simulink model "BackboneTracker"  (R2024b)
settings: Solver=ode4  StartTime=0.0  StopTime=inf  FixedStep=settings.samplingTime_s  MaxStep=1e-2  RelTol=1e-5
PostLoadFcn:
  | , if any(exist('dsrtsu_mdlpostloadfcn', 'file') ~= 0), dsrtsu_mdlpostloadfcn('Execute', bdroot); end,
  | , if any(exist('dsrtsu_mdlpostloadfcn', 'file') ~= 0), dsrtsu_mdlpostloadfcn('Execute', bdroot); end,
InitFcn:
  | , if any(exist('rtifpga_mdlclblib', 'file') ~= 0), rtifpga_mdlclblib('Init', bdroot); end,
values from neighbouring files (symbols this model uses):
  linearModalFrequency_Hz = linearPlantFrequency_Hz    [checkSettingsBackboneTracker.m]
  linearPhiEx = linearPlantPhiEx    [checkSettingsBackboneTracker.m]
undefined symbols (not defined in the file or in its folder): settings
libraries: simulink x8, dspswit3 x4, slpidlib x2, dspsigops x2
settings Model: Tag=RTI1202  DSRTSU_INTERNAL_RTIFPGA=200  DSRTSU_INTERNAL_RTI_TYPE=rti1202  DSRTSU_INTERNAL_RTI_VER=610  RTICANMMDATA=struct('GeneralSetupData',struct('modelroot','C:\UNI\Master\04_MA\05_Experiments','generalsettings',struct('filesettings',struct('destfolder',struct('Name','RTICANMM_FILES','Check',1),'buildfolder',struct('Name','.','Check',1),'AbsDestfolder',struct('Name','C:\UNI\Master\04_MA\05_Experiments\RTICANMM_FILES'),'AbsBuildfolder',struct('Name','C:\UNI\Master\04_MA\05_Experiments'))),'options',struct('addpaths',1,'rmpaths',1,'addtrcexclusion',true,'cannavigator',struct('checkmonitoring',0),'show_usrtrc',0,'use_usrtrc',0),'advanced',struct('options',ones(1,100)),'MPSetup',{{}},'RTI',struct('Type','RTI1202','Ver','7.13','Date','02-Nov-2019'),'modelname','PLL_autoStep_r2019b_rti','block','PLL_autoStep_r2019b_rti'))  DSRTSU_INTERNAL_RTISTBM_VER=22.2  Creator=patri  LastModifiedBy=phippold
settings SolverCC: AlgebraicLoopSolver=TrustRegion
settings DataIOCC: SaveOutput=off  SaveTime=off  ReturnWorkspaceOutputs=off
settings OptimizationCC: BlockReduction=off  OptimizeBlockIOStorage=off  BufferReuse=off  GlobalBufferReuse=off  ExpressionFolding=off  LocalBlockOutputs=off
settings DebuggingCC: UnconnectedInputMsg=warning  UnconnectedOutputMsg=warning  UnconnectedLineMsg=warning  ArithmeticOperatorsInVariantConditions=warning
settings HardwareCC: ProdBitPerPointer=32  ProdBitPerSizeT=32  ProdBitPerPtrDiffT=32  ProdLargestAtomicInteger=Integer  ProdEndianess=BigEndian  ProdWordSize=32  ProdHWDeviceType=Custom Processor->Custom  TargetIntDivRoundTo=Zero  TargetEndianess=BigEndian  TargetHWDeviceType=Custom Processor->Custom
settings ModelReferenceCC: EnableRefExpFcnMdlSchedulingChecks=on  ModelReferenceNumInstancesAllowed=Single  ModelReferenceMinAlgLoopOccurrences=on
settings SFSimCC: SimUseLocalCustomCode=off  MATLABDynamicMemAlloc=off  CustomCodeUndefinedFunction=UseInterfaceOnly
settings RTWCC: Description=dSPACE DS1202 Hardware Platform  SystemTargetFile=rti1202.tlc  MakeCommand=make_rti  TemplateMakefile=rti1202.tmf  RTWUseLocalCustomCode=off  GPUComputeCapability=3.5  DLArmComputeVersion=19.05
settings CodeAppCC: MaxIdLength=63  StateflowObjectComments=on
settings STFCustomTargetCC: ParMdlRefBuildCompliant=on  SystemTargetFile=rti1202.tlc
settings GRTTargetCC: TargetLangStandard=C89/C90 (ANSI)  CompOptLevelCompliant=off  ConcurrentExecutionCompliant=off  CombineOutputUpdateFcns=off  MatFileLogging=off  CPPClassGenCompliant=off  UseToolchainInfoCompliant=off
settings ConfigComp: CovMetricSettings=dswe
settings SimscapeCC: SimscapeNormalizeSystem=off

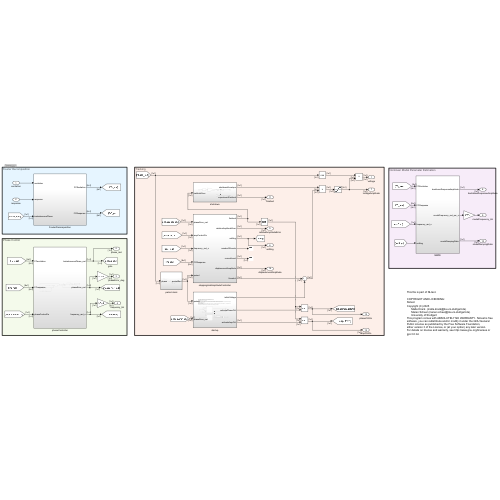
[thumbnail: Simulink's stored preview of the top-level diagram]
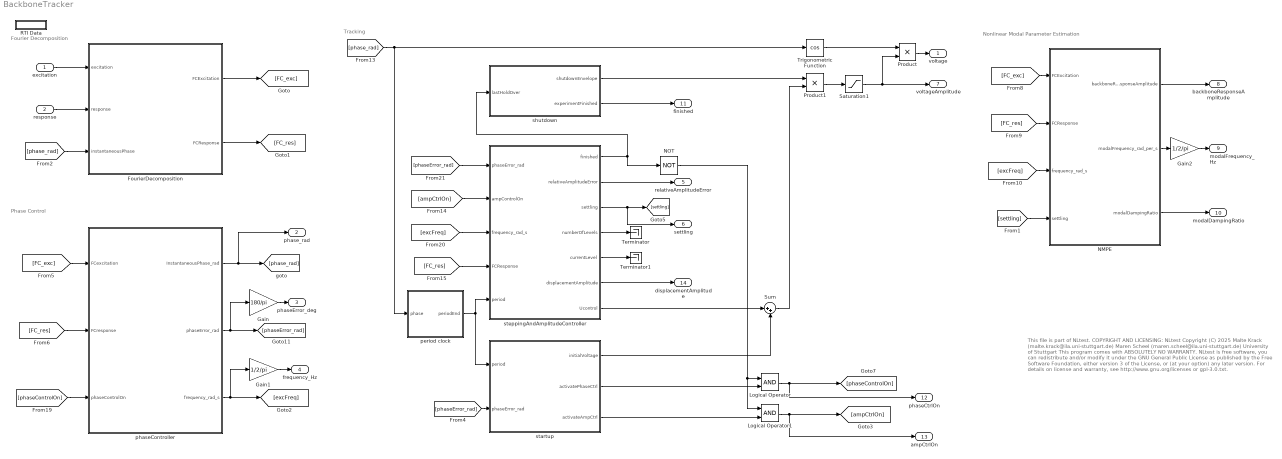
== system BackboneTracker ==
  note: Nonlinear Modal Parameter Estimation
  note: Phase Control
  note: Fourier Decomposition
  note: Tracking
  note: This file is part of NLtest.
      |
      | COPYRIGHT AND LICENSING:
      | NLtest
      | Copyright (C) 2025
      | Malte Krack (malte.krack@ila.uni-stuttgart.de)
      | Maren Scheel (maren.scheel@ila.uni-stuttgart.de)
      | University of Stuttgart
      | This program comes with ABSOLUTELY NO WARRANTY. NLtest is free software, you can redistribute and/or modify it under the GNU General Public License as published by the Free Software Foundation,
      | either version 3 of the License, or (at your option) any later version.
      | For details on license and warranty, see http://www.gnu.org/licenses or gpl-3.0.txt.
  excitation : Inport  OutDataTypeStr=double  PortDimensions=1
  response : Inport  Port=2  OutDataTypeStr=double  PortDimensions=1
  FourierDecomposition : Subsystem
  Gain : Gain  Gain=180/pi
  Gain1 : Gain  Gain=1/2/pi
  Gain2 : Gain  Gain=1/2/pi
  Logical Operator : Logic  AllPortsSameDT=off  OutDataTypeStr=boolean
  Logical Operator1 : Logic  AllPortsSameDT=off  OutDataTypeStr=boolean
  NMPE : Subsystem
  NOT : Logic  Operator=NOT  AllPortsSameDT=off  OutDataTypeStr=boolean
  Product : Product
  Product1 : Product
  RTI Data : Subsystem  Tag=struct('RTIDataServer',struct('RTIDataServerVs','2','RTIModelDescription','struct(''main'',''BackboneTracker_R2022a'',''sub'',''BackboneTracker_R2022a'',''isMp'',0)'))  LoadFcn="if exist('rtidc'), try,  rtidc('DataHostBlockClbLoad', gcbh); catch, disp(['Warning: ''LoadFcn'' for RTI Data block failed: ' lasterr]); end, end,"  mask(RTI_DATA_HOST){}
      mask help:
      | RTI Data Block.
      | This block is used by RTI to store internal model-dependent data.
      | Please keep this block on the root level of the model. Deleting this block will result in data loss.
      |
      | NEVER DELETE OR COPY THIS BLOCK!
      settings: CopyFcn="if exist('rtidc'), try,  rtidc('DataHostBlockClbCopy', gcbh); catch, disp(['Warning: ''CopyFcn'' for RTI Data block failed: ' lasterr]); end, end,"  DeleteFcn="if exist('rtidc'), try,  rtidc('DataHostBlockClbDelete', gcbh); catch, disp(['Warning: ''DeleteFcn'' for RTI Data block failed: ' lasterr]); end, end,"  ModelCloseFcn="if exist('rtidc'), try,  rtidc('DataHostBlockClbModelClose', gcbh); catch, disp(['Warning: ''ModelCloseFcn'' for RTI Data block failed: ' lasterr]); end, end,"  PreSaveFcn="if exist('rtidc'), try,  rtidc('DataHostBlockClbPreSave', gcbh); catch, disp(['Warning: ''PreSaveFcn'' for RTI Data block failed: ' lasterr]); end, end,"  PostSaveFcn="if exist('rtidc'), try,  rtidc('DataHostBlockClbPostSave', gcbh); catch, disp(['Warning: ''PostSaveFcn'' for RTI Data block failed: ' lasterr]); end, end,"  NameChangeFcn="if exist('rtidc'), try,  rtidc('DataHostBlockClbNameChange', gcbh); catch, disp(['Warning: ''NameChangeFcn'' for RTI Data block failed: ' lasterr]); end, end,"
      mask Help:
      | RTI Data Block.
      | This block is used by RTI to store internal model-dependent data.
      | Please keep this block on the root level of the model. Deleting this block will result in data loss.
      | 
      | NEVER DELETE OR COPY THIS BLOCK!
      mask Display:
      | text(0.5, 0.5, 'RTI Data', 'HorizontalAlignment', 'center');
      | plot([1 0]);
  Saturation1 : Saturate  UpperLimit=settings.voltageLimit  LowerLimit=0
  Sum : Sum  Inputs=|++
  Terminator : Terminator
  Terminator1 : Terminator
  Trigonometric Function : Trigonometry  Operator=cos
  period clock : Subsystem
  phaseController : Subsystem
  shutdown : Subsystem
  startup : Subsystem
  steppingAndAmplitudeController : Subsystem
  voltage : Outport  OutDataTypeStr=double  PortDimensions=[1 1]  SampleTime=0
  phase_rad : Outport  Port=2  OutDataTypeStr=double  PortDimensions=[1 1]  SampleTime=0
  phaseError_deg : Outport  Port=3  OutDataTypeStr=double  PortDimensions=[1 1]  SampleTime=0
  frequency_Hz : Outport  Port=4  OutDataTypeStr=double  PortDimensions=[1 1]  SampleTime=0
  relativeAmplitudeError : Outport  Port=5  OutDataTypeStr=double  PortDimensions=[1 1]  SampleTime=0
  settling : Outport  Port=6  OutDataTypeStr=boolean  PortDimensions=[1 1]  SampleTime=[0,1]
  voltageAmplitude : Outport  Port=7  OutDataTypeStr=double  PortDimensions=[1 1]  SampleTime=0
  backboneResponseAmplitude : Outport  Port=8  OutDataTypeStr=double  PortDimensions=[1 1]  SampleTime=0
  modalFrequency_Hz : Outport  Port=9  OutDataTypeStr=double  PortDimensions=1  SampleTime=0
  modalDampingRatio : Outport  Port=10  OutDataTypeStr=double  PortDimensions=[1 1]  SampleTime=0
  finished : Outport  Port=11  OutDataTypeStr=boolean  PortDimensions=[1 1]
  phaseCtrlOn : Outport  Port=12  OutDataTypeStr=boolean  PortDimensions=1
  ampCtrlOn : Outport  Port=13  OutDataTypeStr=boolean  PortDimensions=[1 1]
  displacementAmplitude : Outport  Port=14
  wires:
  [excFreq] -> NMPE/3(frequency_rad_s)
  [phaseError_rad] -> steppingAndAmplitudeController/1(phaseError_rad)
  NMPE/2(modalFrequency_rad_per_s) -> Gain2/1
  [phaseControlOn] -> phaseController/3(phaseControlOn)
  FourierDecomposition/2(FCResponse) -> [FC_res]
  [phase_rad] -> FourierDecomposition/3(instantaneousPhase)
  [phase_rad] -> Trigonometric Function/1, period clock/1(phase)
  [FC_exc] -> phaseController/1(FCexcitation)
  phaseController/2(phaseError_rad) -> Gain/1, [phaseError_rad]
  startup/1(initialVoltage) -> Sum/2
  Product/1 -> voltage/1
  [FC_exc] -> NMPE/1(FCExcitation)
  phaseController/3(frequency_rad_s) -> [excFreq], Gain1/1
  [FC_res] -> phaseController/2(FCresponse)
  [ampCtrlOn] -> steppingAndAmplitudeController/2(ampControlOn)
  steppingAndAmplitudeController/1(finished) -> NOT/1, shutdown/1(lastHoldOver)
  phaseController/1(InstantaneousPhase_rad) -> [phase_rad], phase_rad/1
  steppingAndAmplitudeController/3(settling) -> settling/1, [settling]
  Trigonometric Function/1 -> Product/1
  [excFreq] -> steppingAndAmplitudeController/3(frequency_rad_s)
  period clock/1(periodEnd) -> startup/1(period), steppingAndAmplitudeController/5(period)
  [phaseError_rad] -> startup/2(phaseError_rad)
  NMPE/1(backboneResponseAmplitude) -> backboneResponseAmplitude/1
  [FC_res] -> steppingAndAmplitudeController/4(FCResponse)
  [settling] -> NMPE/4(settling)
  steppingAndAmplitudeController/7(Ucontrol) -> Sum/1
  NMPE/3(modalDampingRatio) -> modalDampingRatio/1
  steppingAndAmplitudeController/2(relativeAmplitudeError) -> relativeAmplitudeError/1
  excitation/1 -> FourierDecomposition/1(excitation)
  response/1 -> FourierDecomposition/2(response)
  FourierDecomposition/1(FCExcitation) -> [FC_exc]
  [FC_res] -> NMPE/2(FCResponse)
  Saturation1/1 -> voltageAmplitude/1, Product/2
  steppingAndAmplitudeController/4(numberOfLevels) -> Terminator/1
  steppingAndAmplitudeController/5(currentLevel) -> Terminator1/1
  startup/2(activatePhaseCtrl) -> Logical Operator/2
  Logical Operator/1 -> phaseCtrlOn/1, [phaseControlOn]
  startup/3(activateAmpCtrl) -> Logical Operator1/2
  Logical Operator1/1 -> [ampCtrlOn], ampCtrlOn/1
  Product1/1 -> Saturation1/1
  Sum/1 -> Product1/2
  shutdown/1(shutdownEnvelope) -> Product1/1
  shutdown/2(experimentFinished) -> finished/1
  NOT/1 -> Logical Operator/1, Logical Operator1/1
  steppingAndAmplitudeController/6(displacementAmplitude) -> displacementAmplitude/1
  Gain/1 -> phaseError_deg/1
  Gain1/1 -> frequency_Hz/1
  Gain2/1 -> modalFrequency_Hz/1

== system BackboneTracker/FourierDecomposition ==
  excitation : Inport
  response : Inport  Port=2
  instantaneousPhase : Inport  Port=3
  Fourier_Decomposition_AF1 : Subsystem  ReferencedSubsystem=Fourier_Decomposition_AF
  Fourier_Decomposition_AF2 : Subsystem  ReferencedSubsystem=Fourier_Decomposition_AF
  FCExcitation : Outport
  FCResponse : Outport  Port=2
  wires:
  Fourier_Decomposition_AF1/1 -> FCResponse/1
  Fourier_Decomposition_AF2/1 -> FCExcitation/1
  response/1 -> Fourier_Decomposition_AF1/1
  instantaneousPhase/1 -> Fourier_Decomposition_AF1/2, Fourier_Decomposition_AF2/2
  excitation/1 -> Fourier_Decomposition_AF2/1

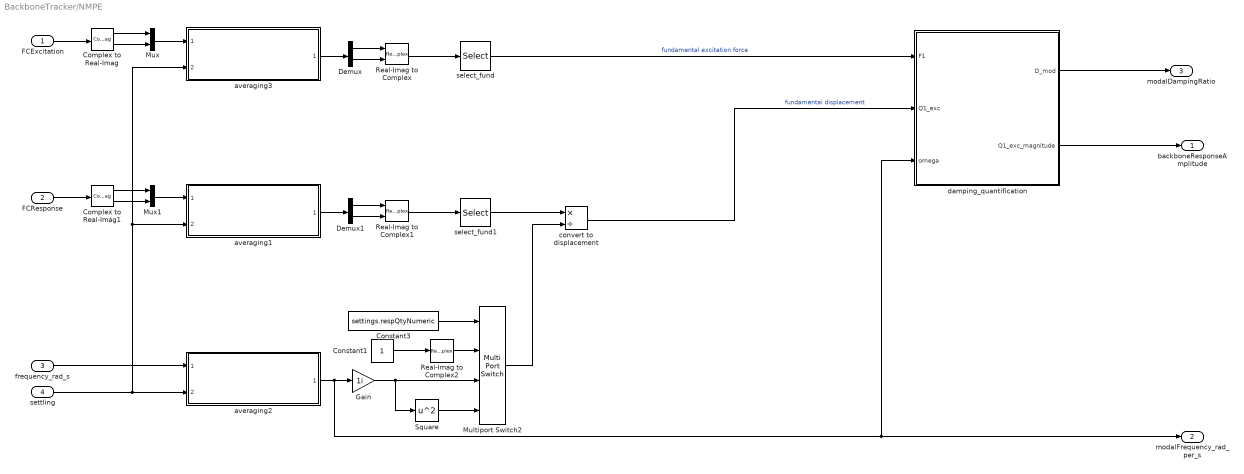
== system BackboneTracker/NMPE ==
  FCExcitation : Inport
  FCResponse : Inport  Port=2
  frequency_rad_s : Inport  Port=3
  settling : Inport  Port=4
  Complex to Real-Imag : ComplexToRealImag
  Complex to Real-Imag1 : ComplexToRealImag
  Constant1 : Constant
  Constant3 : Constant  Value=settings.respQtyNumeric
  Demux : Demux  Outputs=2
  Demux1 : Demux  Outputs=2
  Gain : Gain  Gain=1i
  Multiport Switch2 : MultiPortSwitch  SaturateOnIntegerOverflow=off  InputSameDT=off
  Mux : Mux  Inputs=2
  Mux1 : Mux  Inputs=2
  Real-Imag to Complex : RealImagToComplex
  Real-Imag to Complex1 : RealImagToComplex
  Real-Imag to Complex2 : RealImagToComplex  Input=Real
  Square : Math  Operator=square
  averaging1 : Subsystem  ReferencedSubsystem=Averaging
  averaging2 : Subsystem  ReferencedSubsystem=Averaging
  averaging3 : Subsystem  ReferencedSubsystem=Averaging
  convert to displacement : Product  Inputs=*/
  damping_quantification : Subsystem
  select_fund : Selector  InputPortWidth=settings.H+1  IndexOptions=Index vector (dialog)  Indices=2  OutputSizes=1
  select_fund1 : Selector  InputPortWidth=settings.H+1  IndexOptions=Index vector (dialog)  Indices=2  OutputSizes=1
  backboneResponseAmplitude : Outport
  modalFrequency_rad_per_s : Outport  Port=2
  modalDampingRatio : Outport  Port=3
  wires:
  settling/1 -> averaging1/2, averaging3/2, averaging2/2
  frequency_rad_s/1 -> averaging2/1
  FCExcitation/1 -> Complex to Real-Imag/1
  damping_quantification/1(D_mod) -> modalDampingRatio/1
  averaging2/1 -> Gain/1, damping_quantification/3(omega), modalFrequency_rad_per_s/1
  Constant3/1 -> Multiport Switch2/1
  Real-Imag to Complex2/1 -> Multiport Switch2/2
  Multiport Switch2/1 -> convert to displacement/2
  Square/1 -> Multiport Switch2/4
  Complex to Real-Imag/2 -> Mux/2
  Complex to Real-Imag/1 -> Mux/1
  Demux/1 -> Real-Imag to Complex/1
  Demux/2 -> Real-Imag to Complex/2
  averaging3/1 -> Demux/1
  Mux/1 -> averaging3/1
  Mux1/1 -> averaging1/1
  FCResponse/1 -> Complex to Real-Imag1/1
  Complex to Real-Imag1/2 -> Mux1/2
  Complex to Real-Imag1/1 -> Mux1/1
  Demux1/2 -> Real-Imag to Complex1/2
  Demux1/1 -> Real-Imag to Complex1/1
  averaging1/1 -> Demux1/1
  select_fund/1 -> damping_quantification/1(F1)  "fundamental excitation force"
  Real-Imag to Complex/1 -> select_fund/1
  Real-Imag to Complex1/1 -> select_fund1/1
  select_fund1/1 -> convert to displacement/1
  Gain/1 -> Square/1, Multiport Switch2/3
  convert to displacement/1 -> damping_quantification/2(Q1_exc)  "fundamental displacement"
  Constant1/1 -> Real-Imag to Complex2/1
  damping_quantification/2(Q1_exc_magnitude) -> backboneResponseAmplitude/1

== system BackboneTracker/RTI Data ==
  RTI Data Store : Subsystem  Tag=struct('private',struct('version',struct('dsVer',uint32(2),'dsVerCreation',uint32(2),'RTI',struct('ver','22.2','type','RTI1202')),'access',struct('type','Model','isPerm',1,'created',['02-Jul-2025 10:59:36'],'modified',['16-Jul-2025 13:30:35'],'location','')),'public',struct('main',struct('data',[]),'sub',struct('name','','data',[])))  mask(RTI_DATA_STORE){}
      mask help:
      | RTI Data Store Block. This block is used by RTI to store internal model dependent data. Deleting this block will result in data loss.
      |
      | NEVER DELETE, COPY, OR MODIFY THIS BLOCK!
      mask Help:
      | RTI Data Store Block. This block is used by RTI to store internal model dependent data. Deleting this block will result in data loss.
      | 
      | NEVER DELETE, COPY, OR MODIFY THIS BLOCK!
      mask Display: text(0.5, 0.5, ' ', 'HorizontalAlignment', 'center');

== system BackboneTracker/period clock ==
  note: outputs an impulse every time a period of oscillation has passed
  phase : Inport
  Constant2 : Constant  Value=2*pi
  Divide : Product  Inputs=*/
  Equal : RelationalOperator  Operator=~=  OutDataTypeStr=boolean  RndMeth=Simplest  InputSameDT=off
  Floor : Rounding
  Memory2 : Memory
  periodEnd : Outport
  wires:
  Equal/1 -> periodEnd/1
  Memory2/1 -> Equal/2
  Constant2/1 -> Divide/2
  phase/1 -> Divide/1
  Divide/1 -> Floor/1
  Floor/1 -> Equal/1, Memory2/1

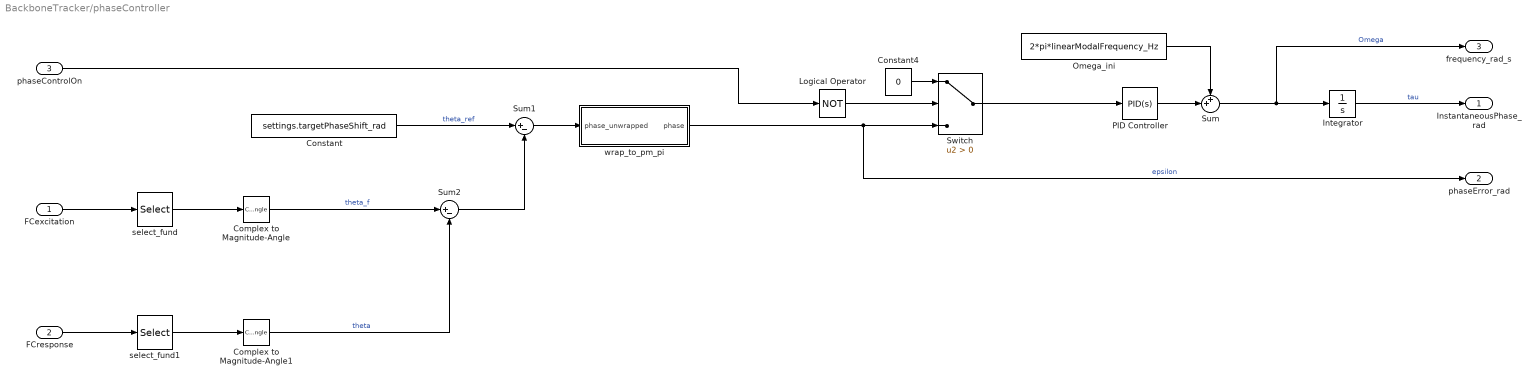
== system BackboneTracker/phaseController ==
  FCexcitation : Inport
  FCresponse : Inport  Port=2
  phaseControlOn : Inport  Port=3
  Complex to Magnitude-Angle : ComplexToMagnitudeAngle  Output=Angle
  Complex to Magnitude-Angle1 : ComplexToMagnitudeAngle  Output=Angle
  Constant : Constant  Value=settings.targetPhaseShift_rad
  Constant4 : Constant  Value=0
  Integrator : Integrator
  Logical Operator : Logic  Operator=NOT  AllPortsSameDT=off  OutDataTypeStr=boolean
  Omega_ini : Constant  Value=2*pi*linearModalFrequency_Hz
  PID Controller : slpidlib/PID Controller  Controller=PID  Form=Parallel  TimeDomain=Continuous-time  UseExternalTs=off  SampleTime=-1  IntegratorMethod=Forward Euler  FilterMethod=Forward Euler  ControllerParametersSource=internal  P=settings.gainsPhaseController.kp  I=settings.gainsPhaseController.ki  UseKiTs=off  D=0  UseExternalDerivativeSource=off  N=100  UseFilter=on  TunerSelectOption=Transfer Function Based (PID Tuner App)  InitialConditionSource=internal  InitialConditionForIntegrator=0  InitialConditionForFilter=0  DifferentiatorICPrevScaledInput=0  ExternalReset=none  TrackingMode=off  Kt=1  LimitOutput=off  SatLimitsSource=internal  UpperSaturationLimit=inf  LowerSaturationLimit=-inf  LinearizeAsGain=on  AntiWindupMode=none  Kb=1  LimitIntegrator=off  UpperIntegratorSaturationLimit=inf  LowerIntegratorSaturationLimit=-inf  POutMin=[]  POutMax=[]  IOutMin=[]  IOutMax=[]  DOutMin=[]  DOutMax=[]  NOutMin=[]  NOutMax=[]  SumOutMin=[]  SumOutMax=[]  SaturationOutMin=[]  SaturationOutMax=[]  PParamMin=[]  PParamMax=[]  IParamMin=[]  IParamMax=[]  DParamMin=[]  DParamMax=[]  NParamMin=[]  NParamMax=[]  KbParamMin=[]  KbParamMax=[]  KtParamMin=[]  KtParamMax=[]  KbOutMin=[]  KbOutMax=[]  KtOutMin=[]  KtOutMax=[]  IntegratorOutMin=[]  IntegratorOutMax=[]  FilterOutMin=[]  FilterOutMax=[]  SumI1OutMin=[]  SumI1OutMax=[]  SumI2OutMin=[]  SumI2OutMax=[]  SumI3OutMin=[]  SumI3OutMax=[]  SumI4OutMin=[]  SumI4OutMax=[]  SumDOutMin=[]  SumDOutMax=[]  DifferentiatorOutMin=[]  DifferentiatorOutMax=[]  FilterDiffOutCoefMin=[]  FilterDiffOutCoefMax=[]  ReciprocalOutMin=[]  ReciprocalOutMax=[]  SumDenOutMin=[]  SumDenOutMax=[]  SumNumOutMin=[]  SumNumOutMax=[]  DivideOutMin=[]  DivideOutMax=[]  UdiffTsProdOutMin=[]  UdiffTsProdOutMax=[]  NTsProdOutMin=[]  NTsProdOutMax=[]  UintegralTsProdOutMin=[]  UintegralTsProdOutMax=[]  UngainTsProdOutMin=[]  UngainTsProdOutMax=[]  ClampingZeroOutDataTypeStr=Inherit: Inherit via back propagation  ClampingZeroOutMin=[]  ClampingZeroOutMax=[]  FilterDenConstantOutDataTypeStr=Inherit: Inherit via back propagation  FilterDenConstantOutMin=[]  FilterDenConstantOutMax=[]  PCopyOutDataTypeStr=Inherit: Inherit via back propagation  PCopyOutMin=[]  PCopyOutMax=[]  NCopyOutDataTypeStr=Inherit: Inherit via back propagation  NCopyOutMin=[]  NCopyOutMax=[]  IntegratorContinuousStateAttributes=''  IntegratorStateMustResolveToSignalObject=off  IntegratorRTWStateStorageClass=Auto  FilterContinuousStateAttributes=''  FilterStateMustResolveToSignalObject=off  FilterRTWStateStorageClass=Auto  ParallelPVariant=InternalParameters  IdealPVariant=Disabled  IVariant=InternalParameters  DVariant=InternalParameters  IntegratorVariant=Continuous  SatVariant=Disabled  AWVariant=Passthrough  PCopyVariant=Disabled  TRVariant=Disabled  FdbkBlocksVariant=Forward  IdealPFdbkVariant=Disabled  SatFdbkVariant=Disabled  DerivativeFilterVariant=ContFilter  NVariant=InternalParameters  NCopyVariant=Disabled  FilterICVariant=InternalICsFilter  IntegratorICVariant=InternalICs  ExternalResetVariant=Disabled  TRSumVariant=Passthrough  SumFdbkVariant=Disabled  SumVariant=Sum_PID  TsampFilterVariant=InternalTs  TsampNgainVariant=Passthrough  TsampIntegralVariant=Disabled_SignalSpec  ExternalSaturationOutDataTypeStr=Inherit: Same as second input  DerivativeSourceVariant=ErrorSignal  PreIntVariant=InternalPreInt
  Sum : Sum  Inputs=++|
  Sum1 : Sum  Inputs=|+-
  Sum2 : Sum  Inputs=|+-
  Switch : Switch  Criteria=u2 > Threshold  SaturateOnIntegerOverflow=off  InputSameDT=off
  select_fund : Selector  InputPortWidth=settings.H+1  IndexOptions=Index vector (dialog)  Indices=2  OutputSizes=1
  select_fund1 : Selector  InputPortWidth=settings.H+1  IndexOptions=Index vector (dialog)  Indices=2  OutputSizes=1
  wrap_to_pm_pi : Subsystem
  InstantaneousPhase_rad : Outport
  phaseError_rad : Outport  Port=2
  frequency_rad_s : Outport  Port=3
  wires:
  Sum2/1 -> Sum1/2
  Sum1/1 -> wrap_to_pm_pi/1(phase_unwrapped)
  Complex to Magnitude-Angle1/1 -> Sum2/2  "theta"
  Complex to Magnitude-Angle/1 -> Sum2/1  "theta_f"
  wrap_to_pm_pi/1(phase) -> phaseError_rad/1, Switch/3  "epsilon"
  Switch/1 -> PID Controller/1
  Constant/1 -> Sum1/1  "theta_ref"
  Integrator/1 -> InstantaneousPhase_rad/1  "tau"
  Omega_ini/1 -> Sum/1
  PID Controller/1 -> Sum/2
  Sum/1 -> Integrator/1, frequency_rad_s/1  "Omega"
  select_fund/1 -> Complex to Magnitude-Angle/1
  FCexcitation/1 -> select_fund/1
  select_fund1/1 -> Complex to Magnitude-Angle1/1
  FCresponse/1 -> select_fund1/1
  Constant4/1 -> Switch/1
  phaseControlOn/1 -> Logical Operator/1
  Logical Operator/1 -> Switch/2

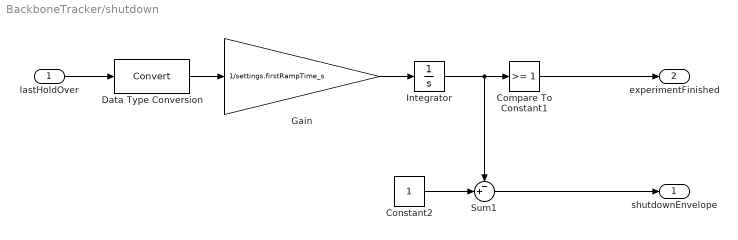
== system BackboneTracker/shutdown ==
  lastHoldOver : Inport
  Compare To Constant1 : simulink/Logic and Bit Operations/Compare To Constant  relop=>=  const=1  OutDataTypeStr=boolean
  Constant2 : Constant
  Data Type Conversion : DataTypeConversion  SaturateOnIntegerOverflow=off  RndMeth=Floor
  Gain : Gain  Gain=1/settings.firstRampTime_s
  Integrator : Integrator
  Sum1 : Sum  Inputs=-+|
  shutdownEnvelope : Outport
  experimentFinished : Outport  Port=2
  wires:
  Constant2/1 -> Sum1/2
  lastHoldOver/1 -> Data Type Conversion/1
  Sum1/1 -> shutdownEnvelope/1
  Compare To Constant1/1 -> experimentFinished/1
  Integrator/1 -> Sum1/1, Compare To Constant1/1
  Data Type Conversion/1 -> Gain/1
  Gain/1 -> Integrator/1

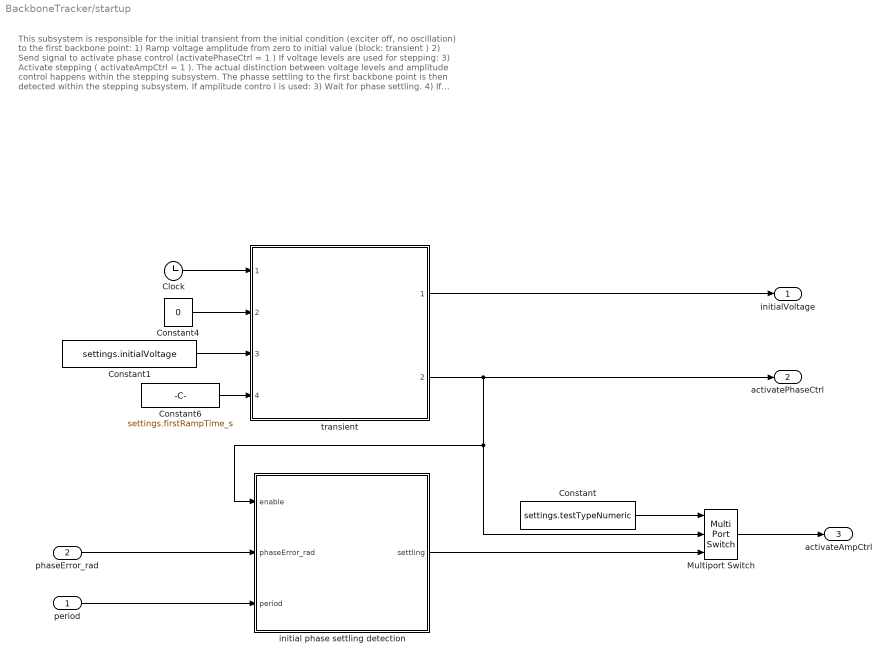
== system BackboneTracker/startup ==
  note: This subsystem is responsible for the initial transient from the initial condition (exciter off, no oscillation) to the first backbone point:
      | 1) Ramp voltage amplitude from zero to initial value (block: transient )
      | 2) Send signal to activate phase control (activatePhaseCtrl = 1 )
      | If voltage levels are used for stepping:
      | 3) Activate stepping ( activateAmpCtrl = 1 ). The actual distinction between voltage levels and amplitude control happens within the stepping subsystem. The phasse settling to the first backbone point is then detected within the stepping subsystem.
      | If amplitude contro l is used:
      | 3) Wait for phase settling.
      | 4) If settling is detected ( initial phase settling detection > settling = 1 ), activate amplitude control ( activateAmpCtrl = 1 ). The amplitude and phase settling to the first backbone point is then detected within the stepping subsystem.
  period : Inport
  phaseError_rad : Inport  Port=2
  Clock : Clock
  Constant : Constant  Value=settings.testTypeNumeric
  Constant1 : Constant  Value=settings.initialVoltage
  Constant4 : Constant  Value=0
  Constant6 : Constant  Value=settings.firstRampTime_s
  Multiport Switch : MultiPortSwitch  Inputs=2  SaturateOnIntegerOverflow=off  InputSameDT=off
  initial phase settling detection : Subsystem
  transient : Subsystem  ReferencedSubsystem=halfCosineRamp
  initialVoltage : Outport
  activatePhaseCtrl : Outport  Port=2
  activateAmpCtrl : Outport  Port=3
  wires:
  Constant/1 -> Multiport Switch/1
  initial phase settling detection/1(settling) -> Multiport Switch/3
  period/1 -> initial phase settling detection/3(period)
  phaseError_rad/1 -> initial phase settling detection/2(phaseError_rad)
  Multiport Switch/1 -> activateAmpCtrl/1
  Constant1/1 -> transient/3
  Constant6/1 -> transient/4
  Constant4/1 -> transient/2
  transient/2 -> activatePhaseCtrl/1, initial phase settling detection/1(enable), Multiport Switch/2
  Clock/1 -> transient/1
  transient/1 -> initialVoltage/1

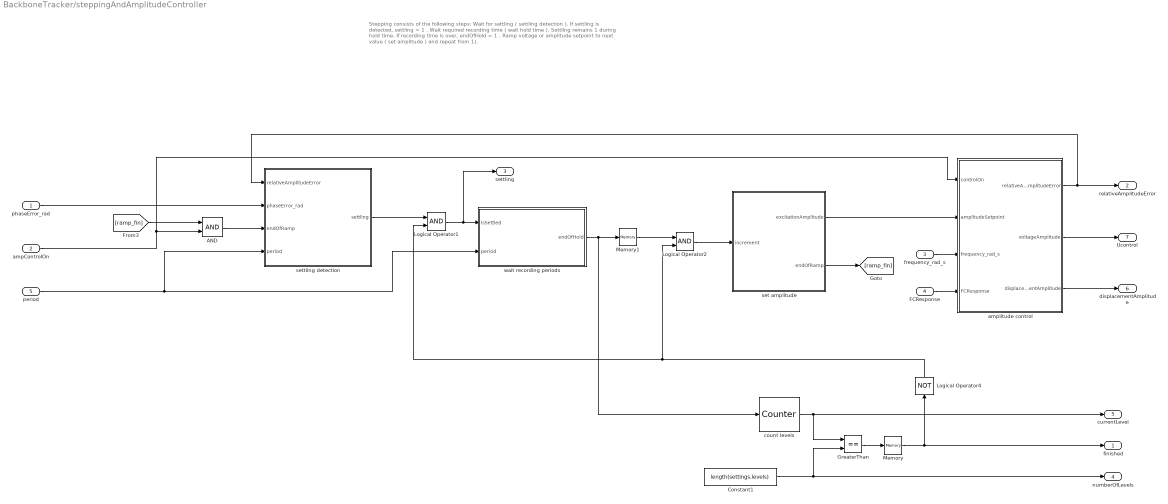
== system BackboneTracker/steppingAndAmplitudeController ==
  note: Stepping consists of the following steps:
      | Wait for settling ( settling detection ). If settling is detected, settling = 1 .
      | Wait required recording time ( wait hold time ). Settling remains 1 during hold time. If recording time is over, endOfHold = 1 .
      | Ramp voltage or amplitude setpoint to next value ( set amplitude ) and repeat from 1).
  phaseError_rad : Inport
  ampControlOn : Inport  Port=2
  frequency_rad_s : Inport  Port=3
  FCResponse : Inport  Port=4
  period : Inport  Port=5
  AND : Logic  AllPortsSameDT=off  OutDataTypeStr=boolean
  Constant1 : Constant  Value=length(settings.levels)
  GreaterThan : RelationalOperator  Operator===  OutDataTypeStr=boolean  RndMeth=Simplest  InputSameDT=off
  Logical Operator1 : Logic  AllPortsSameDT=off  OutDataTypeStr=boolean
  Logical Operator2 : Logic  AllPortsSameDT=off  OutDataTypeStr=boolean
  Logical Operator4 : Logic  Operator=NOT  AllPortsSameDT=off  OutDataTypeStr=boolean
  Memory : Memory
  Memory1 : Memory
  amplitude control : Subsystem
  count levels : dspswit3/Counter  Direction=Up  CountEvent=Rising edge  CounterSize=User defined  MaxCount=4096  InitialCount=0  Output=Count  HitValue=periods_recorded  ResetInput=off  SamplesPerFrame=1  Ts=1  CntDtype=double  HitDtype=Logical
  set amplitude : Subsystem
  settling detection : Subsystem
  wait recording periods : Subsystem
  finished : Outport
  relativeAmplitudeError : Outport  Port=2
  settling : Outport  Port=3
  numberOfLevels : Outport  Port=4
  currentLevel : Outport  Port=5
  displacementAmplitude : Outport  Port=6
  Ucontrol : Outport  Port=7
  wires:
  FCResponse/1 -> amplitude control/4(FCResponse)
  frequency_rad_s/1 -> amplitude control/3(frequency_rad_s)
  amplitude control/2(voltageAmplitude) -> Ucontrol/1
  ampControlOn/1 -> amplitude control/1(controlOn), AND/2
  AND/1 -> settling detection/3(endOfRamp)
  amplitude control/1(relativeAmplitudeError) -> relativeAmplitudeError/1, settling detection/1(relativeAmplitudeError)
  period/1 -> wait recording periods/2(period), settling detection/4(period)
  phaseError_rad/1 -> settling detection/2(phaseError_rad)
  [ramp_fin] -> AND/1
  Logical Operator1/1 -> settling/1, wait recording periods/1(isSettled)
  wait recording periods/1(endOfHold) -> Memory1/1, count levels/1
  set amplitude/2(endOfRamp) -> [ramp_fin]
  set amplitude/1(excitationAmplitude) -> amplitude control/2(amplitudeSetpoint)
  GreaterThan/1 -> Memory/1
  Constant1/1 -> GreaterThan/2, numberOfLevels/1
  count levels/1 -> GreaterThan/1, currentLevel/1
  Memory1/1 -> Logical Operator2/1
  Logical Operator2/1 -> set amplitude/1(increment)
  Memory/1 -> finished/1, Logical Operator4/1
  Logical Operator4/1 -> Logical Operator1/2, Logical Operator2/2
  settling detection/1(settling) -> Logical Operator1/1
  amplitude control/3(displacementAmplitude) -> displacementAmplitude/1

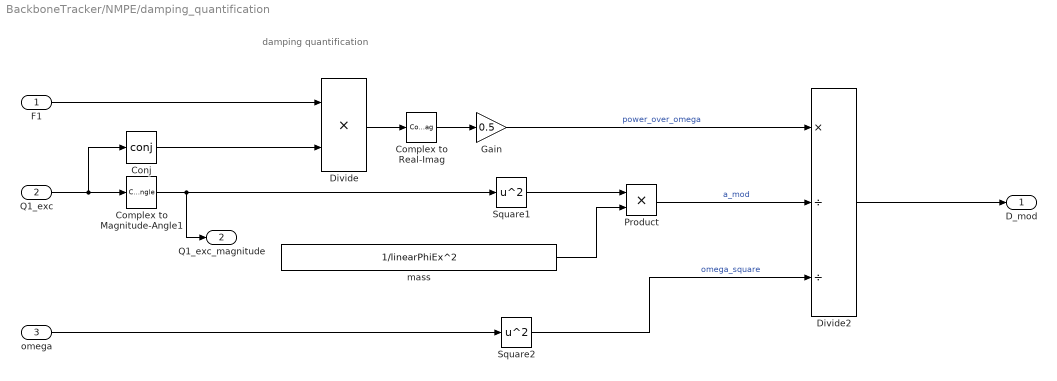
== system BackboneTracker/NMPE/damping_quantification ==
  note: damping quantification
  F1 : Inport
  Q1_exc : Inport  Port=2
  omega : Inport  Port=3
  Complex to Magnitude-Angle1 : ComplexToMagnitudeAngle  Output=Magnitude
  Complex to Real-Imag : ComplexToRealImag  Output=Imag
  Conj : Math  Operator=conj
  Divide : Product  Inputs=**
  Divide2 : Product  Inputs=*//
  Gain : Gain  Gain=0.5
  Product : Product
  Square1 : Math  Operator=square
  Square2 : Math  Operator=square
  mass : Constant  Value=1/linearPhiEx^2
  D_mod : Outport
  Q1_exc_magnitude : Outport  Port=2
  wires:
  Square2/1 -> Divide2/3  "omega_square"
  mass/1 -> Product/2
  Q1_exc/1 -> Conj/1, Complex to Magnitude-Angle1/1
  Square1/1 -> Product/1
  Divide/1 -> Complex to Real-Imag/1
  Product/1 -> Divide2/2  "a_mod"
  F1/1 -> Divide/1
  omega/1 -> Square2/1
  Divide2/1 -> D_mod/1
  Complex to Magnitude-Angle1/1 -> Square1/1, Q1_exc_magnitude/1
  Conj/1 -> Divide/2
  Complex to Real-Imag/1 -> Gain/1
  Gain/1 -> Divide2/1  "power_over_omega"

== system BackboneTracker/RTI Data/RTI Data Store ==
  RTI Data Store : Subsystem  mask(RTI_DATA_STORE){}
      mask help:
      | RTI Data Store Block. This block is used by RTI to store internal model dependent data. Deleting this block will result in data loss.
      |
      | NEVER DELETE, COPY, OR MODIFY THIS BLOCK!
      mask Help:
      | RTI Data Store Block. This block is used by RTI to store internal model dependent data. Deleting this block will result in data loss.
      | 
      | NEVER DELETE, COPY, OR MODIFY THIS BLOCK!
      mask Display: text(0.5, 0.5, ' ', 'HorizontalAlignment', 'center');

== system BackboneTracker/phaseController/wrap_to_pm_pi ==
  phase_unwrapped : Inport
  Trigonometric Function : Trigonometry
  Trigonometric Function1 : Trigonometry  Operator=cos
  Trigonometric Function2 : Trigonometry  Operator=atan2
  phase : Outport
  wires:
  Trigonometric Function2/1 -> phase/1
  Trigonometric Function1/1 -> Trigonometric Function2/2
  Trigonometric Function/1 -> Trigonometric Function2/1
  phase_unwrapped/1 -> Trigonometric Function1/1, Trigonometric Function/1

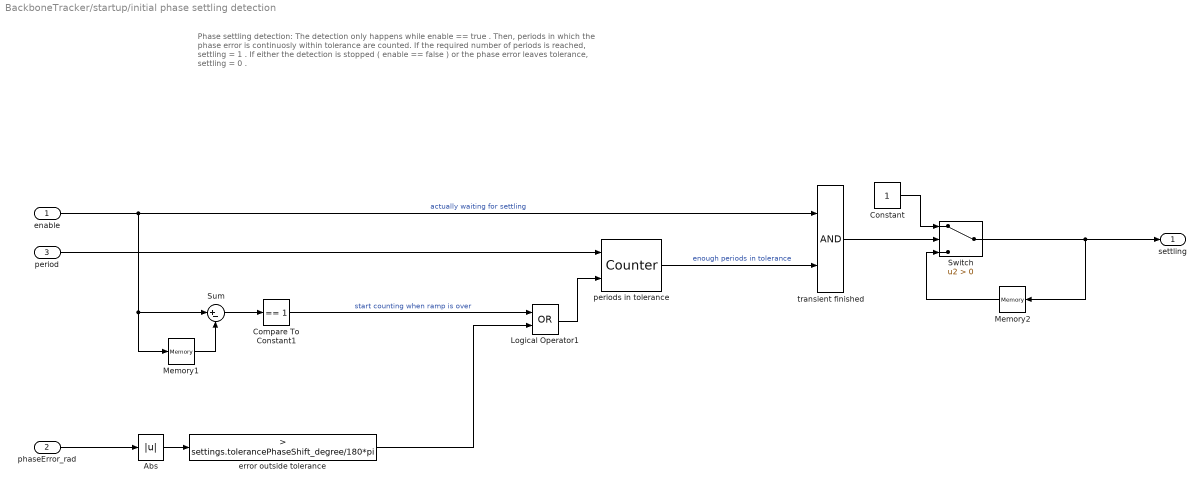
== system BackboneTracker/startup/initial phase settling detection ==
  note: Phase settling detection:
      | The detection only happens while enable == true .
      | Then, periods in which the phase error is continuosly within tolerance are counted.
      | If the required number of periods is reached, settling = 1 .
      | If either the detection is stopped ( enable == false ) or the phase error leaves tolerance, settling = 0 .
  enable : Inport
  phaseError_rad : Inport  Port=2
  period : Inport  Port=3
  Abs : Abs  SaturateOnIntegerOverflow=off
  Compare To Constant1 : simulink/Logic and Bit Operations/Compare To Constant  relop===  const=1  OutDataTypeStr=boolean
  Constant : Constant
  Logical Operator1 : Logic  Operator=OR  AllPortsSameDT=off  OutDataTypeStr=boolean
  Memory1 : Memory
  Memory2 : Memory
  Sum : Sum  Inputs=|+-  OutDataTypeStr=double
  Switch : Switch  Criteria=u2 > Threshold  SaturateOnIntegerOverflow=off  InputSameDT=off
  error outside tolerance : simulink/Logic and Bit Operations/Compare To Constant  relop=>  const=settings.tolerancePhaseShift_degree/180*pi  OutDataTypeStr=boolean
  periods in tolerance : dspswit3/Counter  Direction=Up  CountEvent=Non-zero sample  CounterSize=User defined  MaxCount=settings.periodsInTolerance+1  InitialCount=0  Output=Hit  HitValue=settings.periodsInTolerance+1  ResetInput=on  SamplesPerFrame=1  Ts=1  CntDtype=double  HitDtype=Logical
  transient finished : Logic  AllPortsSameDT=off  OutDataTypeStr=boolean
  settling : Outport
  wires:
  Constant/1 -> Switch/1
  transient finished/1 -> Switch/2
  Memory2/1 -> Switch/3
  Switch/1 -> Memory2/1, settling/1
  phaseError_rad/1 -> Abs/1
  Abs/1 -> error outside tolerance/1
  Memory1/1 -> Sum/2
  Compare To Constant1/1 -> Logical Operator1/1  "start counting when ramp is over"
  Sum/1 -> Compare To Constant1/1
  enable/1 -> Memory1/1, Sum/1, transient finished/1  "actually waiting for settling"
  period/1 -> periods in tolerance/1
  error outside tolerance/1 -> Logical Operator1/2
  Logical Operator1/1 -> periods in tolerance/2
  periods in tolerance/1 -> transient finished/2  "enough periods in tolerance"

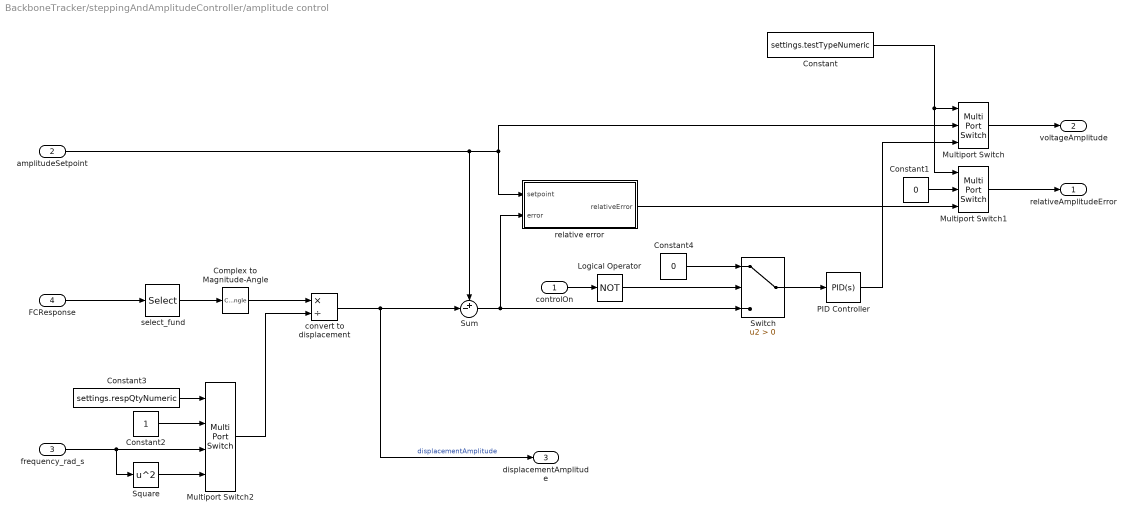
== system BackboneTracker/steppingAndAmplitudeController/amplitude control ==
  controlOn : Inport
  amplitudeSetpoint : Inport  Port=2
  frequency_rad_s : Inport  Port=3
  FCResponse : Inport  Port=4
  Complex to Magnitude-Angle : ComplexToMagnitudeAngle  Output=Magnitude
  Constant : Constant  Value=settings.testTypeNumeric
  Constant1 : Constant  Value=0
  Constant2 : Constant
  Constant3 : Constant  Value=settings.respQtyNumeric
  Constant4 : Constant  Value=0
  Logical Operator : Logic  Operator=NOT  AllPortsSameDT=off  OutDataTypeStr=boolean
  Multiport Switch : MultiPortSwitch  Inputs=2  SaturateOnIntegerOverflow=off  InputSameDT=off
  Multiport Switch1 : MultiPortSwitch  Inputs=2  SaturateOnIntegerOverflow=off  InputSameDT=off
  Multiport Switch2 : MultiPortSwitch  SaturateOnIntegerOverflow=off  InputSameDT=off
  PID Controller : slpidlib/PID Controller  Controller=PID  Form=Parallel  TimeDomain=Continuous-time  UseExternalTs=off  SampleTime=-1  IntegratorMethod=Forward Euler  FilterMethod=Forward Euler  ControllerParametersSource=internal  P=settings.gainsAmplitudeController.kp  I=settings.gainsAmplitudeController.ki  UseKiTs=off  D=0  UseExternalDerivativeSource=off  N=100  UseFilter=on  TunerSelectOption=Transfer Function Based (PID Tuner App)  InitialConditionSource=internal  InitialConditionForIntegrator=0  InitialConditionForFilter=0  DifferentiatorICPrevScaledInput=0  ExternalReset=none  TrackingMode=off  Kt=1  LimitOutput=off  SatLimitsSource=internal  UpperSaturationLimit=inf  LowerSaturationLimit=-inf  LinearizeAsGain=on  AntiWindupMode=none  Kb=1  LimitIntegrator=off  UpperIntegratorSaturationLimit=inf  LowerIntegratorSaturationLimit=-inf  POutMin=[]  POutMax=[]  IOutMin=[]  IOutMax=[]  DOutMin=[]  DOutMax=[]  NOutMin=[]  NOutMax=[]  SumOutMin=[]  SumOutMax=[]  SaturationOutMin=[]  SaturationOutMax=[]  PParamMin=[]  PParamMax=[]  IParamMin=[]  IParamMax=[]  DParamMin=[]  DParamMax=[]  NParamMin=[]  NParamMax=[]  KbParamMin=[]  KbParamMax=[]  KtParamMin=[]  KtParamMax=[]  KbOutMin=[]  KbOutMax=[]  KtOutMin=[]  KtOutMax=[]  IntegratorOutMin=[]  IntegratorOutMax=[]  FilterOutMin=[]  FilterOutMax=[]  SumI1OutMin=[]  SumI1OutMax=[]  SumI2OutMin=[]  SumI2OutMax=[]  SumI3OutMin=[]  SumI3OutMax=[]  SumI4OutMin=[]  SumI4OutMax=[]  SumDOutMin=[]  SumDOutMax=[]  DifferentiatorOutMin=[]  DifferentiatorOutMax=[]  FilterDiffOutCoefMin=[]  FilterDiffOutCoefMax=[]  ReciprocalOutMin=[]  ReciprocalOutMax=[]  SumDenOutMin=[]  SumDenOutMax=[]  SumNumOutMin=[]  SumNumOutMax=[]  DivideOutMin=[]  DivideOutMax=[]  UdiffTsProdOutMin=[]  UdiffTsProdOutMax=[]  NTsProdOutMin=[]  NTsProdOutMax=[]  UintegralTsProdOutMin=[]  UintegralTsProdOutMax=[]  UngainTsProdOutMin=[]  UngainTsProdOutMax=[]  ClampingZeroOutDataTypeStr=Inherit: Inherit via back propagation  ClampingZeroOutMin=[]  ClampingZeroOutMax=[]  FilterDenConstantOutDataTypeStr=Inherit: Inherit via back propagation  FilterDenConstantOutMin=[]  FilterDenConstantOutMax=[]  PCopyOutDataTypeStr=Inherit: Inherit via back propagation  PCopyOutMin=[]  PCopyOutMax=[]  NCopyOutDataTypeStr=Inherit: Inherit via back propagation  NCopyOutMin=[]  NCopyOutMax=[]  IntegratorContinuousStateAttributes=''  IntegratorStateMustResolveToSignalObject=off  IntegratorRTWStateStorageClass=Auto  FilterContinuousStateAttributes=''  FilterStateMustResolveToSignalObject=off  FilterRTWStateStorageClass=Auto  ParallelPVariant=InternalParameters  IdealPVariant=Disabled  IVariant=InternalParameters  DVariant=InternalParameters  IntegratorVariant=Continuous  SatVariant=Disabled  AWVariant=Passthrough  PCopyVariant=Disabled  TRVariant=Disabled  FdbkBlocksVariant=Forward  IdealPFdbkVariant=Disabled  SatFdbkVariant=Disabled  DerivativeFilterVariant=ContFilter  NVariant=InternalParameters  NCopyVariant=Disabled  FilterICVariant=InternalICsFilter  IntegratorICVariant=InternalICs  ExternalResetVariant=Disabled  TRSumVariant=Passthrough  SumFdbkVariant=Disabled  SumVariant=Sum_PID  TsampFilterVariant=InternalTs  TsampNgainVariant=Passthrough  TsampIntegralVariant=Disabled_SignalSpec  ExternalSaturationOutDataTypeStr=Inherit: Same as second input  DerivativeSourceVariant=ErrorSignal  PreIntVariant=InternalPreInt
  Square : Math  Operator=square
  Sum : Sum  Inputs=+-|
  Switch : Switch  Criteria=u2 > Threshold  SaturateOnIntegerOverflow=off  InputSameDT=off
  convert to displacement : Product  Inputs=*/
  relative error : Subsystem  TreatAsAtomicUnit=on
  select_fund : Selector  InputPortWidth=settings.H+1  IndexOptions=Index vector (dialog)  Indices=2  OutputSizes=1
  relativeAmplitudeError : Outport
  voltageAmplitude : Outport  Port=2
  displacementAmplitude : Outport  Port=3
  wires:
  Constant3/1 -> Multiport Switch2/1
  Constant2/1 -> Multiport Switch2/2
  Square/1 -> Multiport Switch2/4
  frequency_rad_s/1 -> Square/1, Multiport Switch2/3
  Multiport Switch2/1 -> convert to displacement/2
  Complex to Magnitude-Angle/1 -> convert to displacement/1
  Constant1/1 -> Multiport Switch1/2
  Multiport Switch1/1 -> relativeAmplitudeError/1
  relative error/1(relativeError) -> Multiport Switch1/3
  PID Controller/1 -> Multiport Switch/3
  Switch/1 -> PID Controller/1
  convert to displacement/1 -> displacementAmplitude/1, Sum/2  "displacementAmplitude"
  Constant/1 -> Multiport Switch/1, Multiport Switch1/1
  Multiport Switch/1 -> voltageAmplitude/1
  amplitudeSetpoint/1 -> Multiport Switch/2, relative error/1(setpoint), Sum/1
  select_fund/1 -> Complex to Magnitude-Angle/1
  FCResponse/1 -> select_fund/1
  Sum/1 -> Switch/3, relative error/2(error)
  controlOn/1 -> Logical Operator/1
  Logical Operator/1 -> Switch/2
  Constant4/1 -> Switch/1

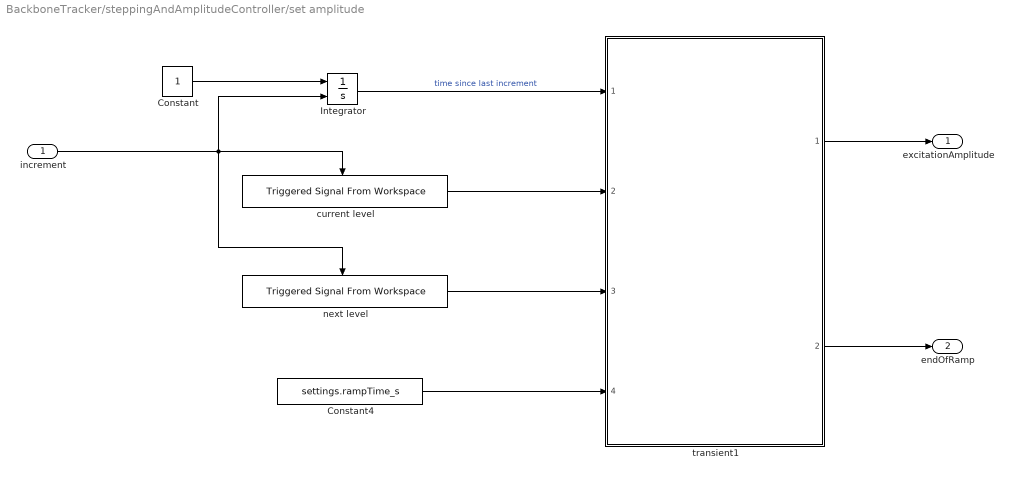
== system BackboneTracker/steppingAndAmplitudeController/set amplitude ==
  increment : Inport
  Constant : Constant
  Constant4 : Constant  Value=settings.rampTime_s
  Integrator : Integrator  ExternalReset=rising
  current level : dspsigops/Triggered Signal From Workspace  Signal=settings.levels(1:end-1)  TriggerType=Rising edge  ic=1e-16  SamplesPerFrame=1  OutputAfterFinalValue=Holding final value  OutputFrames=off
  next level : dspsigops/Triggered Signal From Workspace  Signal=settings.levels(2:end)  TriggerType=Rising edge  ic=settings.levels(1)  SamplesPerFrame=1  OutputAfterFinalValue=Setting to zero  OutputFrames=off
  transient1 : Subsystem  ReferencedSubsystem=halfCosineRamp
  excitationAmplitude : Outport
  endOfRamp : Outport  Port=2
  wires:
  Constant4/1 -> transient1/4
  transient1/2 -> endOfRamp/1
  transient1/1 -> excitationAmplitude/1
  next level/1 -> transient1/3
  Integrator/1 -> transient1/1  "time since last increment"
  Constant/1 -> Integrator/1
  increment/1 -> current level/Trigger, next level/Trigger, Integrator/2
  current level/1 -> transient1/2

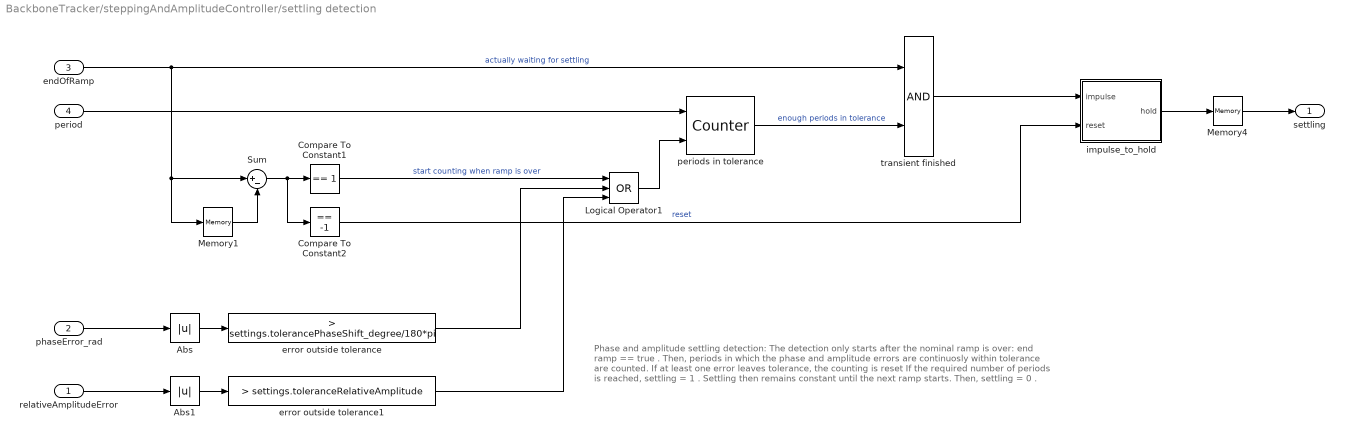
== system BackboneTracker/steppingAndAmplitudeController/settling detection ==
  note: Phase and amplitude settling detection:
      | The detection only starts after the nominal ramp is over: end ramp == true .
      | Then, periods in which the phase and amplitude errors are continuosly within tolerance are counted. If at least one error leaves tolerance, the counting is reset
      | If the required number of periods is reached, settling = 1 .
      | Settling then remains constant until the next ramp starts. Then, settling = 0 .
  relativeAmplitudeError : Inport
  phaseError_rad : Inport  Port=2
  endOfRamp : Inport  Port=3
  period : Inport  Port=4
  Abs : Abs  SaturateOnIntegerOverflow=off
  Abs1 : Abs  SaturateOnIntegerOverflow=off
  Compare To Constant1 : simulink/Logic and Bit Operations/Compare To Constant  relop===  const=1  OutDataTypeStr=boolean
  Compare To Constant2 : simulink/Logic and Bit Operations/Compare To Constant  relop===  const=-1  OutDataTypeStr=boolean
  Logical Operator1 : Logic  Operator=OR  Inputs=3  AllPortsSameDT=off  OutDataTypeStr=boolean
  Memory1 : Memory
  Memory4 : Memory
  Sum : Sum  Inputs=|+-  OutDataTypeStr=double
  error outside tolerance : simulink/Logic and Bit Operations/Compare To Constant  relop=>  const=settings.tolerancePhaseShift_degree/180*pi  OutDataTypeStr=boolean
  error outside tolerance1 : simulink/Logic and Bit Operations/Compare To Constant  relop=>  const=settings.toleranceRelativeAmplitude  OutDataTypeStr=boolean
  impulse_to_hold : Subsystem
  periods in tolerance : dspswit3/Counter  Direction=Up  CountEvent=Non-zero sample  CounterSize=User defined  MaxCount=settings.periodsInTolerance+1  InitialCount=0  Output=Hit  HitValue=settings.periodsInTolerance+1  ResetInput=on  SamplesPerFrame=1  Ts=1  CntDtype=double  HitDtype=Logical
  transient finished : Logic  AllPortsSameDT=off  OutDataTypeStr=boolean
  settling : Outport
  wires:
  impulse_to_hold/1(hold) -> Memory4/1
  Compare To Constant2/1 -> impulse_to_hold/2(reset)  "reset"
  transient finished/1 -> impulse_to_hold/1(impulse)
  Memory4/1 -> settling/1
  relativeAmplitudeError/1 -> Abs1/1
  error outside tolerance1/1 -> Logical Operator1/3
  Abs1/1 -> error outside tolerance1/1
  phaseError_rad/1 -> Abs/1
  Abs/1 -> error outside tolerance/1
  Memory1/1 -> Sum/2
  Compare To Constant1/1 -> Logical Operator1/1  "start counting when ramp is over"
  Sum/1 -> Compare To Constant1/1, Compare To Constant2/1
  endOfRamp/1 -> transient finished/1, Memory1/1, Sum/1  "actually waiting for settling"
  period/1 -> periods in tolerance/1
  error outside tolerance/1 -> Logical Operator1/2
  Logical Operator1/1 -> periods in tolerance/2
  periods in tolerance/1 -> transient finished/2  "enough periods in tolerance"

== system BackboneTracker/steppingAndAmplitudeController/wait recording periods ==
  isSettled : Inport
  period : Inport  Port=2
  Compare To Constant1 : simulink/Logic and Bit Operations/Compare To Constant  relop===  const=1  OutDataTypeStr=boolean
  Counter : dspswit3/Counter  Direction=Up  CountEvent=Non-zero sample  CounterSize=User defined  MaxCount=4096  InitialCount=0  Output=Hit  HitValue=settings.recordedPeriods  ResetInput=on  SamplesPerFrame=1  Ts=1  CntDtype=double  HitDtype=Logical
  Memory1 : Memory
  Sum : Sum  Inputs=|+-  OutDataTypeStr=double
  hold finished : Logic  AllPortsSameDT=off  OutDataTypeStr=boolean
  endOfHold : Outport
  wires:
  period/1 -> Counter/1
  isSettled/1 -> hold finished/1, Sum/1, Memory1/1
  Counter/1 -> hold finished/2
  Sum/1 -> Compare To Constant1/1
  Compare To Constant1/1 -> Counter/2
  hold finished/1 -> endOfHold/1
  Memory1/1 -> Sum/2

== system BackboneTracker/RTI Data/RTI Data Store/RTI Data Store ==
  RTI Data Store : Subsystem  mask(RTI_DATA_STORE){}
      mask help:
      | RTI Data Store Block. This block is used by RTI to store internal model dependent data. Deleting this block will result in data loss.
      |
      | NEVER DELETE, COPY, OR MODIFY THIS BLOCK!
      mask Help:
      | RTI Data Store Block. This block is used by RTI to store internal model dependent data. Deleting this block will result in data loss.
      | 
      | NEVER DELETE, COPY, OR MODIFY THIS BLOCK!
      mask Display: text(0.5, 0.5, ' ', 'HorizontalAlignment', 'center');

== system BackboneTracker/steppingAndAmplitudeController/amplitude control/relative error ==
  note: Divide only if setpoint is greater than zero to avoid error.
  setpoint : Inport
  error : Inport  Port=2
  Constant : Constant
  Divide : Product  Inputs=*/
  Switch : Switch  Criteria=u2 > Threshold  SaturateOnIntegerOverflow=off  InputSameDT=off
  relativeError : Outport
  wires:
  setpoint/1 -> Switch/2, Switch/1
  Divide/1 -> relativeError/1
  Switch/1 -> Divide/2
  error/1 -> Divide/1
  Constant/1 -> Switch/3

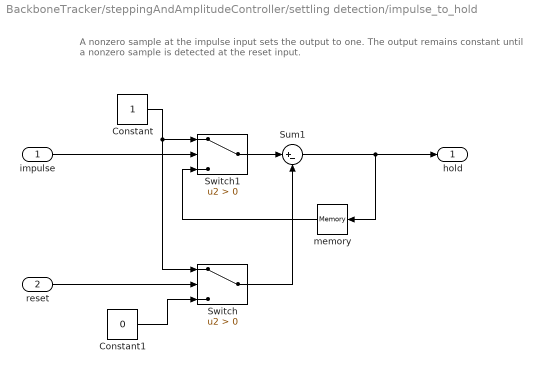
== system BackboneTracker/steppingAndAmplitudeController/settling detection/impulse_to_hold ==
  note: A nonzero sample at the impulse input sets the output to one. The output remains constant until a nonzero sample is detected at the reset input.
  impulse : Inport
  reset : Inport  Port=2
  Constant : Constant
  Constant1 : Constant  Value=0
  Sum1 : Sum  Inputs=|+-
  Switch : Switch  Criteria=u2 > Threshold  SaturateOnIntegerOverflow=off  InputSameDT=off
  Switch1 : Switch  Criteria=u2 > Threshold  SaturateOnIntegerOverflow=off  InputSameDT=off
  memory : Memory
  hold : Outport
  wires:
  impulse/1 -> Switch1/2
  reset/1 -> Switch/2
  Switch/1 -> Sum1/2
  Constant1/1 -> Switch/3
  memory/1 -> Switch1/3
  Switch1/1 -> Sum1/1
  Sum1/1 -> memory/1, hold/1
  Constant/1 -> Switch/1, Switch1/1

== system BackboneTracker/RTI Data/RTI Data Store/RTI Data Store/RTI Data Store ==
  RTI Data Store : Subsystem  mask(RTI_DATA_STORE){}
      mask help:
      | RTI Data Store Block. This block is used by RTI to store internal model dependent data. Deleting this block will result in data loss.
      |
      | NEVER DELETE, COPY, OR MODIFY THIS BLOCK!
      mask Help:
      | RTI Data Store Block. This block is used by RTI to store internal model dependent data. Deleting this block will result in data loss.
      | 
      | NEVER DELETE, COPY, OR MODIFY THIS BLOCK!
      mask Display: text(0.5, 0.5, ' ', 'HorizontalAlignment', 'center');

== system BackboneTracker/RTI Data/RTI Data Store/RTI Data Store/RTI Data Store/RTI Data Store ==
